simulink model "siso"  (R2021a)
settings: Solver=FixedStepDiscrete  StartTime=0.0  StopTime=2  FixedStep=1/16000  RelTol=1e-3
libraries: dspsrcs4 x1, dspvision x1, simulink x1
settings Model: Creator=gonze  LastModifiedBy=chuid
settings SolverCC: AlgebraicLoopSolver=TrustRegion
settings DebuggingCC: SFMachineParentedDataDiag=warning

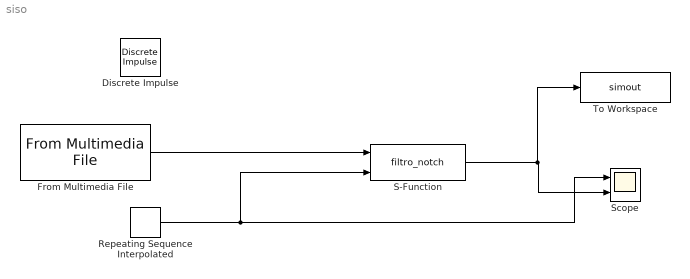
== system siso ==
  Discrete Impulse : dspsrcs4/Discrete  Impulse  Delay=0  SampleTime=0.01  FrameSample=1  OutputFrames=off  dataType=double  isSigned=on  wordLen=16  udDataType=sfix(16)  fracBitsMode=Best precision  numFracBits=15  OutDataTypeStr=double  LastOutDataTypeStr=double
  From Multimedia File : dspvision/From Multimedia File  inputFilename=C:\Users\chuid\Documents\GitHub\LabDSP-Repositorio\lab3dsp_G7_Aguilera_Huidobro\alternate_tones_16_16.wav  readRange=[1 Inf]  loop=on  numPlays=inf  outputStreams=Audio only  videoDataType=single  audioDataType=double  inheritSampleTime=on  userDefinedSampleTime=1/30  noAudioOutput=off  isIntensityVideo=off  fourcc=RGB  colorVideoFormat=Separate color signals  outputEOF=off  dataOrg=Column-major  audioFrameSize=1  computeAudioFrameSize=off  outSamplingMode=Sample based
  Repeating Sequence Interpolated : simulink/Sources/Repeating Sequence Interpolated  OutValues=[440 440 880 880].'  TimeValues="[0  0.2 1.8 2].'"  LookUpMeth=Interpolation-Use End Values  tsamp=0.01  OutMin=[]  OutMax=[]  OutDataTypeStr=double  OutputDataTypeScalingMode=double  OutDataType=fixdt(0,8)  OutScaling=2^-10
  S-Function : S-Function  FunctionName=filtro_notch  SFunctionDeploymentMode=off  EnableBusSupport=off
  Scope : Scope  NumInputPorts=2
  To Workspace : ToWorkspace  VariableName=simout  SampleTime=-1
      settings: Save2DSignal=2-D array (concatenate along first dimension)
  wires:
  S-Function/1 -> To Workspace/1, Scope/2
  Repeating Sequence Interpolated/1 -> Scope/1, S-Function/2
  From Multimedia File/1 -> S-Function/1
